simulink model "Final_System_Model_V10"  (R2018a)
settings: Solver=VariableStepAuto  StartTime=0  StopTime=250  FixedStep=0.5  RelTol=1e-3
PreLoadFcn:
  | Ts_Power=1e-6;
  | Ts_Control=100e-6;
undefined symbols (not defined in the file): DiscIntNeverNeededParam, sigbuilder_block
libraries: simulink x24, fl_lib x16, powerlib x15, nesl_utility x8, powerlib_meascontrol x5, re_lib x1
(part 7 of 8)

== system Final_System_Model_V10/Full System/Subsystem1/100KW Fuel Cell Stack_2/Fuel Cell Model/ From Current Density (A//cm^2) To Overvoltages (V)/Activation Overvoltage ==
  note: % Activation Losses
      | b = R .*Tk./(2 .*Alpha .*F);
      | V_act = -b .*log(i./io) % Tafel equation
  Temperature/C1 : Inport
  Current Density (i)(A/cm^2) : Inport  Port=2
  Add : Sum
  Alpha Charge Transfer Coefficient1 : Constant  Value=Alpha_charge_Transfer_Coefficient
  Bus Creator : BusCreator  Inputs=6
  Bus Creator1 : BusCreator  Inputs=3
  Bus Selector : BusSelector  OutputSignals=8:314,Stack Temperature (C),273:15,2,Faraday Constant,Alpha
  Bus Selector1 : BusSelector  OutputSignals=b,Current Density (A/cm^2),i_0
  Constant : Constant  Value=273.15
  Constant1 : Constant  Value=8.314
  Constant2 : Constant  Value=2
  Divide : Product  Inputs=*/
  Farady Constant : Constant  Value=96485
  Gain : Gain  Gain=-1
  Math Function : Math  Operator=log10  SaturateOnIntegerOverflow=on
  Product : Product  Inputs=3
  Product1 : Product
  Product2 : Product
  Reference Exchange Current Density (I_0)1 : Constant  Value=Exchange_Current_Density_i0
  b : Product  Inputs=*/
  Activation Overvoltage1 (V) : Outport
  Exchange Current Density (i_0) : Outport  Port=2
  wires:
  Alpha Charge Transfer Coefficient1/1 -> Bus Creator/2  "Alpha"
  Temperature/C1/1 -> Bus Creator/1
  Current Density (i)(A/cm^2)/1 -> Bus Creator1/2
  Reference Exchange Current Density (I_0)1/1 -> Bus Creator1/3, Exchange Current Density (i_0)/1  "i_0"
  Product2/1 -> Activation Overvoltage1 (V)/1  "Activation Overvoltage"
  Bus Creator/1 -> Bus Selector/1
  Constant/1 -> Bus Creator/3  "273:15"
  Constant1/1 -> Bus Creator/4  "8:314"
  Farady Constant/1 -> Bus Creator/5  "Faraday Constant"
  Constant2/1 -> Bus Creator/6  "2"
  Bus Selector/4 -> Product/1  "<2>"
  Bus Selector/5 -> Product/2  "<Faraday Constant>"
  Bus Selector/6 -> Product/3  "<Alpha>"
  Product/1 -> b/2
  Bus Selector/1 -> Product1/1  "<8:314>"
  Bus Selector/2 -> Add/1  "<Stack Temperature (C)>"
  Bus Selector/3 -> Add/2  "<273:15>"
  Add/1 -> Product1/2  "Temperature/K"
  Product1/1 -> b/1
  b/1 -> Bus Creator1/1  "b"
  Bus Creator1/1 -> Bus Selector1/1
  Bus Selector1/1 -> Gain/1  "<b>"
  Bus Selector1/2 -> Divide/1  "<Current Density (A/cm^2)>"
  Bus Selector1/3 -> Divide/2  "<i_0>"
  Gain/1 -> Product2/1
  Divide/1 -> Math Function/1
  Math Function/1 -> Product2/2

== system Final_System_Model_V10/Full System/Subsystem1/100KW Fuel Cell Stack_2/Fuel Cell Model/ From Current Density (A//cm^2) To Overvoltages (V)/Concentration Overvoltage ==
  note: V_conc = Alpha1 .*(i.^k) .*log(1-(i./il));
      | term=1-(i/i_l)
  Current Density (i)1 : Inport
  Add : Sum  Inputs=+-
  Amplification Constant Alpha2 : Constant  Value=Amplification_Constant_Alpha1
  Bus Creator : BusCreator  Inputs=3
  Bus Creator1 : BusCreator  Inputs=4
  Bus Selector : BusSelector  OutputSignals=1,Current Density (i),Limiting Current Density (i_L)
  Bus Selector1 : BusSelector  OutputSignals=Amplification Constant(Alpha1),Current Density (i),Mass Transport Limit (K),ln term
  Constant : Constant
  Constant1 : Constant  Value=0.01
  Constant2 : Constant  Value=0
  Divide : Product  Inputs=*/
  IF Function : Subsystem
  Limiting Current (i_L)1 : Constant  Value=Limiting_Current_Density_i_l
  Mass Transport Constant (K)1 : Constant  Value=Mass_Transport_Limit_k
  Math Function1 : Math  Operator=pow  SaturateOnIntegerOverflow=on
  Product : Product  Inputs=3
  Saturation Dynamic : simulink/Discontinuities/Saturation Dynamic  OutMin=[]  OutMax=[]  OutDataTypeStr=Inherit: Same as second input  OutDataType=fixdt(1, 16)  OutScaling=2^-10  DoSatur=off
  Subtract : Sum  Inputs=+-
  "Concentration Overvoltage1 (V) " : Outport
  wires:
  Bus Creator/1 -> Bus Selector/1
  Limiting Current (i_L)1/1 -> Subtract/1, Bus Creator/2  "Limiting Current Density (i_L)"
  Saturation Dynamic/1 -> Bus Creator1/1, Bus Creator/1  "Current Density (i)"
  Mass Transport Constant (K)1/1 -> Bus Creator1/2  "Mass Transport Limit (K)"
  Amplification Constant Alpha2/1 -> Bus Creator1/4  "Amplification Constant(Alpha1)"
  Product/1 -> "Concentration Overvoltage1 (V) "/1  "Concentration Overvoltage"
  Constant/1 -> Bus Creator/3  "1"
  Bus Selector/1 -> Add/1  "<1>"
  Bus Selector/2 -> Divide/1  "<Current Density (i)>"
  Bus Selector/3 -> Divide/2  "<Limiting Current Density (i_L)>"
  Divide/1 -> Add/2
  Add/1 -> IF Function/1(In1)
  IF Function/1(Out1) -> Bus Creator1/3  "ln term"
  Bus Creator1/1 -> Bus Selector1/1
  Bus Selector1/1 -> Product/1  "<Amplification Constant(Alpha1)>"
  Bus Selector1/2 -> Math Function1/1  "<Current Density (i)>"
  Bus Selector1/3 -> Math Function1/2  "<Mass Transport Limit (K)>"
  Bus Selector1/4 -> Product/3  "<ln term>"
  Math Function1/1 -> Product/2
  Current Density (i)1/1 -> Saturation Dynamic/2  "Current Density (i)"
  Constant1/1 -> Subtract/2
  Subtract/1 -> Saturation Dynamic/1
  Constant2/1 -> Saturation Dynamic/3

== system Final_System_Model_V10/Full System/Subsystem1/100KW Fuel Cell Stack_2/Fuel Cell Model/ From Current Density (A//cm^2) To Overvoltages (V)/Ohmic Overvoltage ==
  Current Density (i ) : Inport
  Constant : Constant  Value=-1
  Internal Resistance (r) : Constant  Value=Internal_Resistance_r
  V_Resistive1 : Product  Inputs=3
  V_Resistive : Outport
  wires:
  Constant/1 -> V_Resistive1/3
  Internal Resistance (r)/1 -> V_Resistive1/2
  Current Density (i )/1 -> V_Resistive1/1
  V_Resistive1/1 -> V_Resistive/1  "Ohmic Overvoltage (V)"

== system Final_System_Model_V10/Full System/Subsystem1/100KW Fuel Cell Stack_2/Fuel Cell Model/Air Flow Rate To Current (A)/From Stack Current (A) To Oxygen Mass Flow Rate(kg//s) ==
  Current (A) : Inport
  Number Of Cells : Inport  Port=2
  Divide : Product  Inputs=*/
  F : Constant  Value=96487
  Oxygen Molar Mass (Kg/mol) : Constant  Value=32e-3
  Product : Product
  Product1 : Product
  Product2 : Product
  c : Constant  Value=4
  Oxygen Flow Rate (kg/s) : Outport
  wires:
  F/1 -> Product1/1
  Current (A)/1 -> Product/1
  Product/1 -> Divide/1
  Oxygen Molar Mass (Kg/mol)/1 -> Product2/2
  c/1 -> Product1/2
  Divide/1 -> Product2/1
  Product1/1 -> Divide/2
  Product2/1 -> Oxygen Flow Rate (kg/s)/1
  Number Of Cells/1 -> Product/2

== system Final_System_Model_V10/Full System/Subsystem1/100KW Fuel Cell Stack_2/Fuel Cell Model/From Mass Flow Rates (kg//s) To Current Density (A//cm^2)/From Current (A) To Current Density (A//cm^2) ==
  note: i=I/A
      | where i=Current Density (A/cm^2)
      | I= Current (A)
      | A=Cell Area (cm^2)
  Nominal Current (A) : Inport
  Cell Area (cm^2) : Inport  Port=2
  Divide : Product  Inputs=*/
  Current Density (A/cm^2) : Outport
  wires:
  Nominal Current (A)/1 -> Divide/1
  Cell Area (cm^2)/1 -> Divide/2
  Divide/1 -> Current Density (A/cm^2)/1

== system Final_System_Model_V10/Full System/Subsystem1/100KW Fuel Cell Stack_2/Fuel Cell Model/From Mass Flow Rates (kg//s) To Current Density (A//cm^2)/Fuel Mass Flow Rate (kg//s) To Current (A) ==
  note: This block calculates the output Current (A) from the Hydrogen Mass Flow Rate (kg/s)
      | I=Hydrogen Mass Flow Rate (kg/s)*2*F/(M_H2*n)
      | where: I=Current (A)
      | F=Faraday Constant=96487 C/mol
      | M_H2=hydrogen molar mass=2.016*10^-3 kg/mol
      | n=Number of Cells
  Hydrogen Flow Rate (kg/s) : Inport
  Number Of Cells : Inport  Port=2
  Constant1 : Constant  Value=2
  Divide : Product  Inputs=*/
  F : Constant  Value=96487
  Hydrogen Molar Mass : Constant  Value=2.016e-3
  Product : Product
  Product1 : Product
  Product2 : Product
  Current (A) : Outport
  wires:
  F/1 -> Product1/2
  Constant1/1 -> Product1/1
  Product1/1 -> Product/2
  Product/1 -> Divide/1
  Hydrogen Molar Mass/1 -> Product2/1
  Number Of Cells/1 -> Product2/2
  Product2/1 -> Divide/2
  Divide/1 -> Current (A)/1
  Hydrogen Flow Rate (kg/s)/1 -> Product/1

== system Final_System_Model_V10/Full System/Subsystem1/100KW Fuel Cell Stack_2/Fuel Cell Model/From Pressures (atm) To Nernest Voltage (V)/From Absolute Pressure (atm) To Partial Pressures (atm) ==
  Current Density (i ) : Inport
  Hydrogen Pressure (P_H2) : Inport  Port=2
  Air Pressure (P_air) : Inport  Port=3
  Temperature/C : Inport  Port=4
  Bus Creator : BusCreator  Inputs=5
  Bus Selector : BusSelector  OutputSignals=Air Pressure (atm),Stack Temperature (C),Current Density (A/cm^2),Water Pressure(atm)
  Bus Selector1 : BusSelector  OutputSignals=Stack Temperature (C)
  Bus Selector2 : BusSelector  OutputSignals=Hydrogen Pressure (atm),Stack Temperature (C),Current Density (A/cm^2),Water Pressure(atm)
  Hydrogen Partial Pressure Output : Subsystem
  Oxygen Partial Pressure Output : Subsystem
  Water Pressure output : Subsystem
  Hydrogen Partial Pressure (pp_H2) : Outport
  Oxygen Partial Pressure pp_O2 : Outport  Port=2
  Water Pressure : Outport  Port=3
  wires:
  Water Pressure output/1(Water Pressure) -> Water Pressure/1, Bus Creator/3
  Air Pressure (P_air)/1 -> Bus Creator/1
  Oxygen Partial Pressure Output/1(Oxygen Partial Pressure pp_O2) -> Oxygen Partial Pressure pp_O2/1
  Hydrogen Partial Pressure Output/1(Hydrogen Partial Pressure (pp_H2)) -> Hydrogen Partial Pressure (pp_H2)/1
  Current Density (i )/1 -> Bus Creator/2  "Current Density (A/cm^2)"
  Temperature/C/1 -> Bus Creator/4
  Hydrogen Pressure (P_H2)/1 -> Bus Creator/5
  Bus Creator/1 -> Bus Selector2/1, Bus Selector/1, Bus Selector1/1
  Bus Selector/1 -> Oxygen Partial Pressure Output/1(Air Pressure (P_air))  "<Air Pressure (atm)>"
  Bus Selector/2 -> Oxygen Partial Pressure Output/2(Temperature/C)  "<Stack Temperature (C)>"
  Bus Selector/3 -> Oxygen Partial Pressure Output/3(Current Density/i)  "<Current Density (A/cm^2)>"
  Bus Selector/4 -> Oxygen Partial Pressure Output/4(Water Pressure)  "<Water Pressure(atm)>"
  Bus Selector1/1 -> Water Pressure output/1(Temperature/C)  "<Stack Temperature (C)>"
  Bus Selector2/1 -> Hydrogen Partial Pressure Output/1(Hydrogen Pressure (P_H2))  "<Hydrogen Pressure (atm)>"
  Bus Selector2/2 -> Hydrogen Partial Pressure Output/2(Temperature/C)  "<Stack Temperature (C)>"
  Bus Selector2/3 -> Hydrogen Partial Pressure Output/3(Current Density (i ))  "<Current Density (A/cm^2)>"
  Bus Selector2/4 -> Hydrogen Partial Pressure Output/4(Water Pressure)  "<Water Pressure(atm)>"

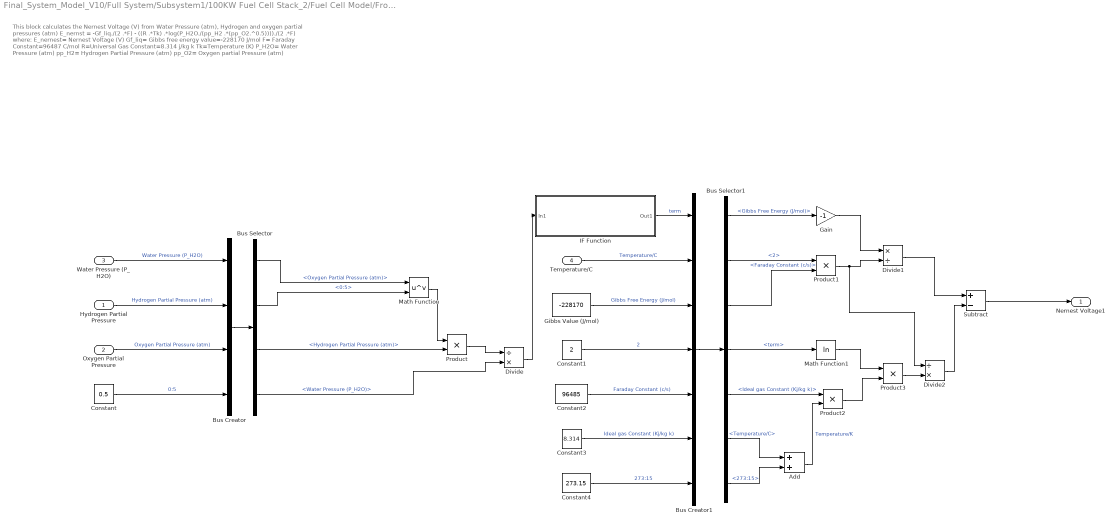
== system Final_System_Model_V10/Full System/Subsystem1/100KW Fuel Cell Stack_2/Fuel Cell Model/From Pressures (atm) To Nernest Voltage (V)/From Partial Pressures (atm) To Nernest Voltage (V) ==
  note: This block calculates the Nernest Voltage (V) from Water Pressure (atm), Hydrogen and oxygen partial pressures (atm)
      | E_nernst = -Gf_liq./(2 .*F) - ((R .*Tk) .*log(P_H2O./(pp_H2 .*(pp_O2.^0.5))))./(2 .*F)
      | where: E_nernest= Nernest Voltage (V)
      | Gf_liq= Gibbs free energy value=-228170 J/mol
      | F= Faraday Constant=96487 C/mol
      | R=Universal Gas Constant=8.314 j/kg k
      | Tk=Temperature (K)
      | P_H2O= Water Pressure (atm)
      | pp_H2= Hydrogen Partial Pressure (atm)
      | pp_O2= Oxygen partial Pressure (atm)
  Hydrogen Partial Pressure : Inport
  Oxygen Partial Pressure : Inport  Port=2
  Water Pressure (P_H2O) : Inport  Port=3
  Temperature/C : Inport  Port=4
  Add : Sum
  Bus Creator : BusCreator  Inputs=4
  Bus Creator1 : BusCreator  Inputs=7
  Bus Selector : BusSelector  OutputSignals=Oxygen Partial Pressure (atm),0:5,Hydrogen Partial Pressure (atm),Water Pressure (P_H2O)
  Bus Selector1 : BusSelector  OutputSignals=Gibbs Free Energy (J/mol),2,Faraday Constant (c/s),term,Ideal gas Constant (Kj/kg k),Temperature/C,273:15
  Constant : Constant  Value=0.5
  Constant1 : Constant  Value=2
  Constant2 : Constant  Value=96485
  Constant3 : Constant  Value=8.314
  Constant4 : Constant  Value=273.15
  Divide : Product  Inputs=/*
  Divide1 : Product  Inputs=*/
  Divide2 : Product  Inputs=/*
  Gain : Gain  Gain=-1
  Gibbs Value (J/mol) : Constant  Value=-228170
  IF Function : Subsystem
  Math Function : Math  Operator=pow  SaturateOnIntegerOverflow=on
  Math Function1 : Math  Operator=log  SaturateOnIntegerOverflow=on
  Product{,1..3} (4 alike) : Product
  Subtract : Sum  Inputs=+-
  Nernest Voltage1 : Outport
  wires:
  Gibbs Value (J/mol)/1 -> Bus Creator1/3  "Gibbs Free Energy (J/mol)"
  Oxygen Partial Pressure/1 -> Bus Creator/3  "Oxygen Partial Pressure (atm)"
  Water Pressure (P_H2O)/1 -> Bus Creator/1  "Water Pressure (P_H2O)"
  Hydrogen Partial Pressure/1 -> Bus Creator/2  "Hydrogen Partial Pressure (atm)"
  Temperature/C/1 -> Bus Creator1/2  "Temperature/C"
  Bus Creator/1 -> Bus Selector/1
  Bus Selector/2 -> Math Function/2  "<0:5>"
  Constant/1 -> Bus Creator/4  "0:5"
  Bus Selector/1 -> Math Function/1  "<Oxygen Partial Pressure (atm)>"
  Bus Selector/3 -> Product/2  "<Hydrogen Partial Pressure (atm)>"
  Math Function/1 -> Product/1
  Bus Selector/4 -> Divide/2  "<Water Pressure (P_H2O)>"
  Product/1 -> Divide/1
  Divide/1 -> IF Function/1(In1)
  IF Function/1(Out1) -> Bus Creator1/1  "term"
  Bus Creator1/1 -> Bus Selector1/1
  Constant1/1 -> Bus Creator1/4  "2"
  Constant2/1 -> Bus Creator1/5  "Faraday Constant (c/s)"
  Bus Selector1/1 -> Gain/1  "<Gibbs Free Energy (J/mol)>"
  Gain/1 -> Divide1/1
  Bus Selector1/2 -> Product1/1  "<2>"
  Bus Selector1/3 -> Product1/2  "<Faraday Constant (c/s)>"
  Product1/1 -> Divide2/1, Divide1/2
  Divide1/1 -> Subtract/1
  Bus Selector1/4 -> Math Function1/1  "<term>"
  Math Function1/1 -> Product3/1
  Constant3/1 -> Bus Creator1/6  "Ideal gas Constant (Kj/kg k)"
  Constant4/1 -> Bus Creator1/7  "273:15"
  Bus Selector1/5 -> Product2/1  "<Ideal gas Constant (Kj/kg k)>"
  Bus Selector1/6 -> Add/1  "<Temperature/C>"
  Bus Selector1/7 -> Add/2  "<273:15>"
  Add/1 -> Product2/2  "Temperature/K"
  Product2/1 -> Product3/2
  Product3/1 -> Divide2/2
  Divide2/1 -> Subtract/2
  Subtract/1 -> Nernest Voltage1/1

== system Final_System_Model_V10/Full System/Subsystem1/80KW Fuel Cell Stack_1/Fuel Cell Model/ From Current Density (A//cm^2) To Overvoltages (V)/Activation Overvoltage ==
  note: % Activation Losses
      | b = R .*Tk./(2 .*Alpha .*F);
      | V_act = -b .*log(i./io) % Tafel equation
  Temperature/C1 : Inport
  Current Density (i)(A/cm^2) : Inport  Port=2
  Add : Sum
  Alpha Charge Transfer Coefficient1 : Constant  Value=Alpha_charge_Transfer_Coefficient
  Bus Creator : BusCreator  Inputs=6
  Bus Creator1 : BusCreator  Inputs=3
  Bus Selector : BusSelector  OutputSignals=8:314,Stack Temperature (C),273:15,2,Faraday Constant,Alpha
  Bus Selector1 : BusSelector  OutputSignals=b,Current Density (A/cm^2),i_0
  Constant : Constant  Value=273.15
  Constant1 : Constant  Value=8.314
  Constant2 : Constant  Value=2
  Divide : Product  Inputs=*/
  Farady Constant : Constant  Value=96485
  Gain : Gain  Gain=-1
  Math Function : Math  Operator=log10  SaturateOnIntegerOverflow=on
  Product : Product  Inputs=3
  Product1 : Product
  Product2 : Product
  Reference Exchange Current Density (I_0)1 : Constant  Value=Exchange_Current_Density_i0
  b : Product  Inputs=*/
  Activation Overvoltage1 (V) : Outport
  Exchange Current Density (i_0) : Outport  Port=2
  wires:
  Math Function/1 -> Product2/2
  Divide/1 -> Math Function/1
  Gain/1 -> Product2/1
  Bus Selector1/3 -> Divide/2  "<i_0>"
  Bus Selector1/2 -> Divide/1  "<Current Density (A/cm^2)>"
  Bus Selector1/1 -> Gain/1  "<b>"
  Bus Creator1/1 -> Bus Selector1/1
  b/1 -> Bus Creator1/1  "b"
  Product1/1 -> b/1
  Add/1 -> Product1/2  "Temperature/K"
  Bus Selector/3 -> Add/2  "<273:15>"
  Bus Selector/2 -> Add/1  "<Stack Temperature (C)>"
  Bus Selector/1 -> Product1/1  "<8:314>"
  Product/1 -> b/2
  Bus Selector/6 -> Product/3  "<Alpha>"
  Bus Selector/5 -> Product/2  "<Faraday Constant>"
  Bus Selector/4 -> Product/1  "<2>"
  Constant2/1 -> Bus Creator/6  "2"
  Farady Constant/1 -> Bus Creator/5  "Faraday Constant"
  Constant1/1 -> Bus Creator/4  "8:314"
  Constant/1 -> Bus Creator/3  "273:15"
  Bus Creator/1 -> Bus Selector/1
  Product2/1 -> Activation Overvoltage1 (V)/1  "Activation Overvoltage"
  Reference Exchange Current Density (I_0)1/1 -> Exchange Current Density (i_0)/1, Bus Creator1/3  "i_0"
  Current Density (i)(A/cm^2)/1 -> Bus Creator1/2
  Temperature/C1/1 -> Bus Creator/1
  Alpha Charge Transfer Coefficient1/1 -> Bus Creator/2  "Alpha"

== system Final_System_Model_V10/Full System/Subsystem1/80KW Fuel Cell Stack_1/Fuel Cell Model/ From Current Density (A//cm^2) To Overvoltages (V)/Concentration Overvoltage ==
  note: V_conc = Alpha1 .*(i.^k) .*log(1-(i./il));
      | term=1-(i/i_l)
  Current Density (i)1 : Inport
  Add : Sum  Inputs=+-
  Amplification Constant Alpha2 : Constant  Value=Amplification_Constant_Alpha1
  Bus Creator : BusCreator  Inputs=3
  Bus Creator1 : BusCreator  Inputs=4
  Bus Selector : BusSelector  OutputSignals=1,Current Density (i),Limiting Current Density (i_L)
  Bus Selector1 : BusSelector  OutputSignals=Amplification Constant(Alpha1),Current Density (i),Mass Transport Limit (K),ln term
  Constant : Constant
  Constant1 : Constant  Value=0.01
  Constant2 : Constant  Value=0
  Divide : Product  Inputs=*/
  IF Function : Subsystem
  Limiting Current (i_L)1 : Constant  Value=Limiting_Current_Density_i_l
  Mass Transport Constant (K)1 : Constant  Value=Mass_Transport_Limit_k
  Math Function1 : Math  Operator=pow  SaturateOnIntegerOverflow=on
  Product : Product  Inputs=3
  Saturation Dynamic : simulink/Discontinuities/Saturation Dynamic  OutMin=[]  OutMax=[]  OutDataTypeStr=Inherit: Same as second input  OutDataType=fixdt(1, 16)  OutScaling=2^-10  DoSatur=off
  Subtract : Sum  Inputs=+-
  "Concentration Overvoltage1 (V) " : Outport
  wires:
  Constant2/1 -> Saturation Dynamic/3
  Subtract/1 -> Saturation Dynamic/1
  Constant1/1 -> Subtract/2
  Current Density (i)1/1 -> Saturation Dynamic/2  "Current Density (i)"
  Math Function1/1 -> Product/2
  Bus Selector1/4 -> Product/3  "<ln term>"
  Bus Selector1/3 -> Math Function1/2  "<Mass Transport Limit (K)>"
  Bus Selector1/2 -> Math Function1/1  "<Current Density (i)>"
  Bus Selector1/1 -> Product/1  "<Amplification Constant(Alpha1)>"
  Bus Creator1/1 -> Bus Selector1/1
  IF Function/1(Out1) -> Bus Creator1/3  "ln term"
  Add/1 -> IF Function/1(In1)
  Divide/1 -> Add/2
  Bus Selector/3 -> Divide/2  "<Limiting Current Density (i_L)>"
  Bus Selector/2 -> Divide/1  "<Current Density (i)>"
  Bus Selector/1 -> Add/1  "<1>"
  Constant/1 -> Bus Creator/3  "1"
  Product/1 -> "Concentration Overvoltage1 (V) "/1  "Concentration Overvoltage"
  Amplification Constant Alpha2/1 -> Bus Creator1/4  "Amplification Constant(Alpha1)"
  Mass Transport Constant (K)1/1 -> Bus Creator1/2  "Mass Transport Limit (K)"
  Saturation Dynamic/1 -> Bus Creator/1, Bus Creator1/1  "Current Density (i)"
  Limiting Current (i_L)1/1 -> Bus Creator/2, Subtract/1  "Limiting Current Density (i_L)"
  Bus Creator/1 -> Bus Selector/1

== system Final_System_Model_V10/Full System/Subsystem1/80KW Fuel Cell Stack_1/Fuel Cell Model/ From Current Density (A//cm^2) To Overvoltages (V)/Ohmic Overvoltage ==
  Current Density (i ) : Inport
  Constant : Constant  Value=-1
  Internal Resistance (r) : Constant  Value=Internal_Resistance_r
  V_Resistive1 : Product  Inputs=3
  V_Resistive : Outport
  wires:
  V_Resistive1/1 -> V_Resistive/1  "Ohmic Overvoltage (V)"
  Current Density (i )/1 -> V_Resistive1/1
  Internal Resistance (r)/1 -> V_Resistive1/2
  Constant/1 -> V_Resistive1/3

== system Final_System_Model_V10/Full System/Subsystem1/80KW Fuel Cell Stack_1/Fuel Cell Model/Air Flow Rate To Current (A)/From Stack Current (A) To Oxygen Mass Flow Rate(kg//s) ==
  Current (A) : Inport
  Number Of Cells : Inport  Port=2
  Divide : Product  Inputs=*/
  F : Constant  Value=96487
  Oxygen Molar Mass (Kg/mol) : Constant  Value=32e-3
  Product : Product
  Product1 : Product
  Product2 : Product
  c : Constant  Value=4
  Oxygen Flow Rate (kg/s) : Outport
  wires:
  Number Of Cells/1 -> Product/2
  Product2/1 -> Oxygen Flow Rate (kg/s)/1
  Product1/1 -> Divide/2
  Divide/1 -> Product2/1
  c/1 -> Product1/2
  Oxygen Molar Mass (Kg/mol)/1 -> Product2/2
  Product/1 -> Divide/1
  Current (A)/1 -> Product/1
  F/1 -> Product1/1

== system Final_System_Model_V10/Full System/Subsystem1/80KW Fuel Cell Stack_1/Fuel Cell Model/From Mass Flow Rates (kg//s) To Current Density (A//cm^2)/From Current (A) To Current Density (A//cm^2) ==
  note: i=I/A
      | where i=Current Density (A/cm^2)
      | I= Current (A)
      | A=Cell Area (cm^2)
  Nominal Current (A) : Inport
  Cell Area (cm^2) : Inport  Port=2
  Divide : Product  Inputs=*/
  Current Density (A/cm^2) : Outport
  wires:
  Divide/1 -> Current Density (A/cm^2)/1
  Cell Area (cm^2)/1 -> Divide/2
  Nominal Current (A)/1 -> Divide/1

== system Final_System_Model_V10/Full System/Subsystem1/80KW Fuel Cell Stack_1/Fuel Cell Model/From Mass Flow Rates (kg//s) To Current Density (A//cm^2)/Fuel Mass Flow Rate (kg//s) To Current (A) ==
  note: This block calculates the output Current (A) from the Hydrogen Mass Flow Rate (kg/s)
      | I=Hydrogen Mass Flow Rate (kg/s)*2*F/(M_H2*n)
      | where: I=Current (A)
      | F=Faraday Constant=96487 C/mol
      | M_H2=hydrogen molar mass=2.016*10^-3 kg/mol
      | n=Number of Cells
  Hydrogen Flow Rate (kg/s) : Inport
  Number Of Cells : Inport  Port=2
  Constant1 : Constant  Value=2
  Divide : Product  Inputs=*/
  F : Constant  Value=96487
  Hydrogen Molar Mass : Constant  Value=2.016e-3
  Product : Product
  Product1 : Product
  Product2 : Product
  Current (A) : Outport
  wires:
  Hydrogen Flow Rate (kg/s)/1 -> Product/1
  Divide/1 -> Current (A)/1
  Product2/1 -> Divide/2
  Number Of Cells/1 -> Product2/2
  Hydrogen Molar Mass/1 -> Product2/1
  Product/1 -> Divide/1
  Product1/1 -> Product/2
  Constant1/1 -> Product1/1
  F/1 -> Product1/2

== system Final_System_Model_V10/Full System/Subsystem1/80KW Fuel Cell Stack_1/Fuel Cell Model/From Pressures (atm) To Nernest Voltage (V)/From Absolute Pressure (atm) To Partial Pressures (atm) ==
  Current Density (i ) : Inport
  Hydrogen Pressure (P_H2) : Inport  Port=2
  Air Pressure (P_air) : Inport  Port=3
  Temperature/C : Inport  Port=4
  Bus Creator : BusCreator  Inputs=5
  Bus Selector : BusSelector  OutputSignals=Air Pressure (atm),Stack Temperature (C),Current Density (A/cm^2),Water Pressure(atm)
  Bus Selector1 : BusSelector  OutputSignals=Stack Temperature (C)
  Bus Selector2 : BusSelector  OutputSignals=Hydrogen Pressure (atm),Stack Temperature (C),Current Density (A/cm^2),Water Pressure(atm)
  Hydrogen Partial Pressure Output : Subsystem
  Oxygen Partial Pressure Output : Subsystem
  Water Pressure output : Subsystem
  Hydrogen Partial Pressure (pp_H2) : Outport
  Oxygen Partial Pressure pp_O2 : Outport  Port=2
  Water Pressure : Outport  Port=3
  wires:
  Bus Selector2/4 -> Hydrogen Partial Pressure Output/4(Water Pressure)  "<Water Pressure(atm)>"
  Bus Selector2/3 -> Hydrogen Partial Pressure Output/3(Current Density (i ))  "<Current Density (A/cm^2)>"
  Bus Selector2/2 -> Hydrogen Partial Pressure Output/2(Temperature/C)  "<Stack Temperature (C)>"
  Bus Selector2/1 -> Hydrogen Partial Pressure Output/1(Hydrogen Pressure (P_H2))  "<Hydrogen Pressure (atm)>"
  Bus Selector1/1 -> Water Pressure output/1(Temperature/C)  "<Stack Temperature (C)>"
  Bus Selector/4 -> Oxygen Partial Pressure Output/4(Water Pressure)  "<Water Pressure(atm)>"
  Bus Selector/3 -> Oxygen Partial Pressure Output/3(Current Density/i)  "<Current Density (A/cm^2)>"
  Bus Selector/2 -> Oxygen Partial Pressure Output/2(Temperature/C)  "<Stack Temperature (C)>"
  Bus Selector/1 -> Oxygen Partial Pressure Output/1(Air Pressure (P_air))  "<Air Pressure (atm)>"
  Bus Creator/1 -> Bus Selector1/1, Bus Selector/1, Bus Selector2/1
  Hydrogen Pressure (P_H2)/1 -> Bus Creator/5
  Temperature/C/1 -> Bus Creator/4
  Current Density (i )/1 -> Bus Creator/2  "Current Density (A/cm^2)"
  Hydrogen Partial Pressure Output/1(Hydrogen Partial Pressure (pp_H2)) -> Hydrogen Partial Pressure (pp_H2)/1
  Oxygen Partial Pressure Output/1(Oxygen Partial Pressure pp_O2) -> Oxygen Partial Pressure pp_O2/1
  Air Pressure (P_air)/1 -> Bus Creator/1
  Water Pressure output/1(Water Pressure) -> Bus Creator/3, Water Pressure/1

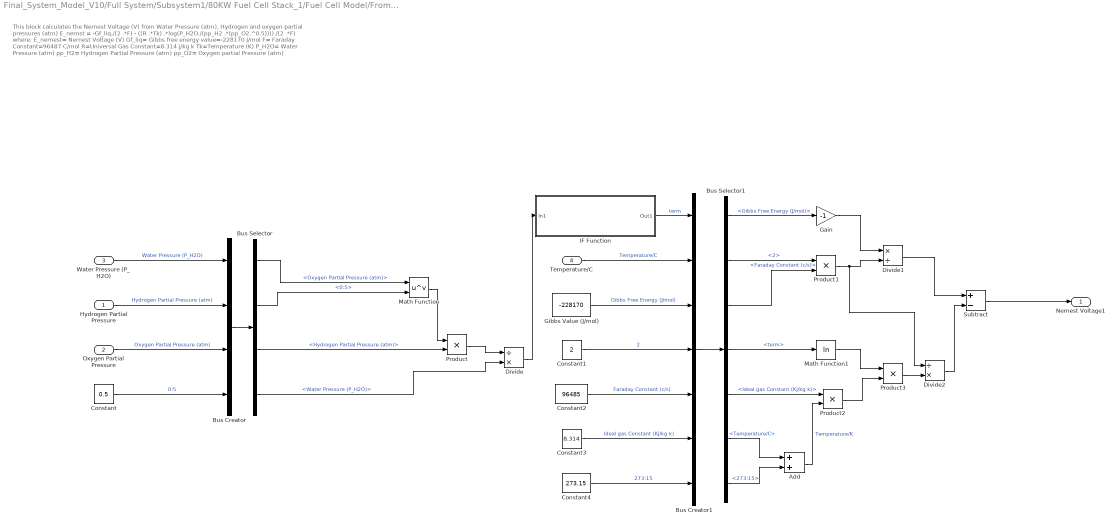
== system Final_System_Model_V10/Full System/Subsystem1/80KW Fuel Cell Stack_1/Fuel Cell Model/From Pressures (atm) To Nernest Voltage (V)/From Partial Pressures (atm) To Nernest Voltage (V) ==
  note: This block calculates the Nernest Voltage (V) from Water Pressure (atm), Hydrogen and oxygen partial pressures (atm)
      | E_nernst = -Gf_liq./(2 .*F) - ((R .*Tk) .*log(P_H2O./(pp_H2 .*(pp_O2.^0.5))))./(2 .*F)
      | where: E_nernest= Nernest Voltage (V)
      | Gf_liq= Gibbs free energy value=-228170 J/mol
      | F= Faraday Constant=96487 C/mol
      | R=Universal Gas Constant=8.314 j/kg k
      | Tk=Temperature (K)
      | P_H2O= Water Pressure (atm)
      | pp_H2= Hydrogen Partial Pressure (atm)
      | pp_O2= Oxygen partial Pressure (atm)
  Hydrogen Partial Pressure : Inport
  Oxygen Partial Pressure : Inport  Port=2
  Water Pressure (P_H2O) : Inport  Port=3
  Temperature/C : Inport  Port=4
  Add : Sum
  Bus Creator : BusCreator  Inputs=4
  Bus Creator1 : BusCreator  Inputs=7
  Bus Selector : BusSelector  OutputSignals=Oxygen Partial Pressure (atm),0:5,Hydrogen Partial Pressure (atm),Water Pressure (P_H2O)
  Bus Selector1 : BusSelector  OutputSignals=Gibbs Free Energy (J/mol),2,Faraday Constant (c/s),term,Ideal gas Constant (Kj/kg k),Temperature/C,273:15
  Constant : Constant  Value=0.5
  Constant1 : Constant  Value=2
  Constant2 : Constant  Value=96485
  Constant3 : Constant  Value=8.314
  Constant4 : Constant  Value=273.15
  Divide : Product  Inputs=/*
  Divide1 : Product  Inputs=*/
  Divide2 : Product  Inputs=/*
  Gain : Gain  Gain=-1
  Gibbs Value (J/mol) : Constant  Value=-228170
  IF Function : Subsystem
  Math Function : Math  Operator=pow  SaturateOnIntegerOverflow=on
  Math Function1 : Math  Operator=log  SaturateOnIntegerOverflow=on
  Product{,1..3} (4 alike) : Product
  Subtract : Sum  Inputs=+-
  Nernest Voltage1 : Outport
  wires:
  Subtract/1 -> Nernest Voltage1/1
  Divide2/1 -> Subtract/2
  Product3/1 -> Divide2/2
  Product2/1 -> Product3/2
  Add/1 -> Product2/2  "Temperature/K"
  Bus Selector1/7 -> Add/2  "<273:15>"
  Bus Selector1/6 -> Add/1  "<Temperature/C>"
  Bus Selector1/5 -> Product2/1  "<Ideal gas Constant (Kj/kg k)>"
  Constant4/1 -> Bus Creator1/7  "273:15"
  Constant3/1 -> Bus Creator1/6  "Ideal gas Constant (Kj/kg k)"
  Math Function1/1 -> Product3/1
  Bus Selector1/4 -> Math Function1/1  "<term>"
  Divide1/1 -> Subtract/1
  Product1/1 -> Divide1/2, Divide2/1
  Bus Selector1/3 -> Product1/2  "<Faraday Constant (c/s)>"
  Bus Selector1/2 -> Product1/1  "<2>"
  Gain/1 -> Divide1/1
  Bus Selector1/1 -> Gain/1  "<Gibbs Free Energy (J/mol)>"
  Constant2/1 -> Bus Creator1/5  "Faraday Constant (c/s)"
  Constant1/1 -> Bus Creator1/4  "2"
  Bus Creator1/1 -> Bus Selector1/1
  IF Function/1(Out1) -> Bus Creator1/1  "term"
  Divide/1 -> IF Function/1(In1)
  Product/1 -> Divide/1
  Bus Selector/4 -> Divide/2  "<Water Pressure (P_H2O)>"
  Math Function/1 -> Product/1
  Bus Selector/3 -> Product/2  "<Hydrogen Partial Pressure (atm)>"
  Bus Selector/1 -> Math Function/1  "<Oxygen Partial Pressure (atm)>"
  Constant/1 -> Bus Creator/4  "0:5"
  Bus Selector/2 -> Math Function/2  "<0:5>"
  Bus Creator/1 -> Bus Selector/1
  Temperature/C/1 -> Bus Creator1/2  "Temperature/C"
  Hydrogen Partial Pressure/1 -> Bus Creator/2  "Hydrogen Partial Pressure (atm)"
  Water Pressure (P_H2O)/1 -> Bus Creator/1  "Water Pressure (P_H2O)"
  Oxygen Partial Pressure/1 -> Bus Creator/3  "Oxygen Partial Pressure (atm)"
  Gibbs Value (J/mol)/1 -> Bus Creator1/3  "Gibbs Free Energy (J/mol)"

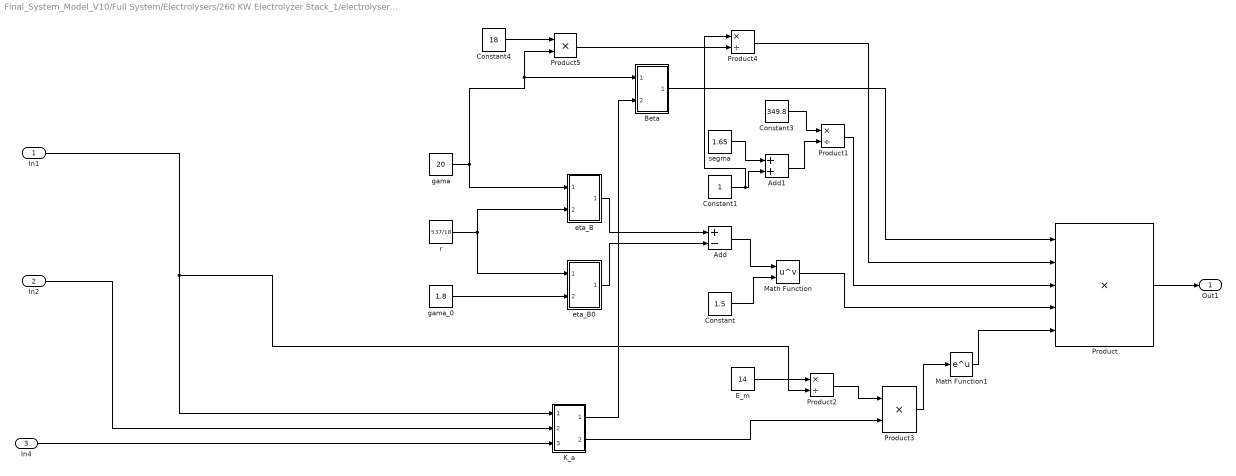
== system Final_System_Model_V10/Full System/Electrolysers/260 KW Electrolyzer Stack_1/electrolyser stack/electrolyser cell/Eta_B/segma_B ==
  In1 : Inport
  In2 : Inport  Port=2
  In4 : Inport  Port=3
  Add : Sum  Inputs=+-
  Add1 : Sum
  Beta : Subsystem
  Constant : Constant  Value=1.5
  Constant1 : Constant
  Constant3 : Constant  Value=349.8
  Constant4 : Constant  Value=18
  E_m : Constant  Value=14
  K_a : Subsystem
  Math Function : Math  Operator=pow  SaturateOnIntegerOverflow=on
  Math Function1 : Math  SaturateOnIntegerOverflow=on
  Product : Product  Inputs=5
  Product1 : Product  Inputs=*/
  Product2 : Product  Inputs=*/
  Product3 : Product
  Product4 : Product  Inputs=*/
  Product5 : Product  Inputs=**
  eta_B : Subsystem
  eta_B0 : Subsystem
  gama : Constant  Value=20
  gama_0 : Constant  Value=1.8
  r : Constant  Value=537/18
  segma : Constant  Value=1.65
  Out1 : Outport
  wires:
  Constant1/1 -> Product4/1, Add1/2
  Math Function1/1 -> Product/5
  eta_B0/1(Out1) -> Add/2
  In4/1 -> K_a/3(In3)
  In1/1 -> Product2/2, K_a/1(In1)
  In2/1 -> K_a/2(In2)
  Product5/1 -> Product4/2
  K_a/1(Out1) -> Beta/2(In2)
  Constant3/1 -> Product1/1
  Math Function/1 -> Product/4
  E_m/1 -> Product2/1
  Constant/1 -> Math Function/2
  Add1/1 -> Product1/2
  segma/1 -> Add1/1
  Product1/1 -> Product/3
  gama_0/1 -> eta_B0/2(In2)
  Product3/1 -> Math Function1/1
  Add/1 -> Math Function/1
  Beta/1(Out1) -> Product/1
  Constant4/1 -> Product5/1
  Product4/1 -> Product/2
  gama/1 -> Product5/2, Beta/1(In1), eta_B/1(In1)
  r/1 -> eta_B0/1(In1), eta_B/2(In2)
  Product/1 -> Out1/1
  eta_B/1(Out1) -> Add/1
  K_a/2(Out2) -> Product3/2
  Product2/1 -> Product3/1

== system Final_System_Model_V10/Full System/Electrolysers/260 KW Electrolyzer Stack_1/electrolyser stack/electrolyser cell/eta_a/m_a ==
  In1 : Inport
  Constant : Constant
  Divide : Product  Inputs=*/
  Subtract : Sum  Inputs=+-
  limiting current : Constant  Value=2
  Out1 : Outport
  wires:
  In1/1 -> Divide/1
  limiting current/1 -> Divide/2
  Constant/1 -> Subtract/1
  Subtract/1 -> Out1/1
  Divide/1 -> Subtract/2

== system Final_System_Model_V10/Full System/Electrolysers/260 KW Electrolyzer Stack_1/electrolyser stack/electrolyser cell/eta_a/n_a ==
  In1 : Inport
  In2 : Inport  Port=2
  In3 : Inport  Port=3
  Divide : Product  Inputs=*/
  i_a0 : Subsystem
  Out1 : Outport
  wires:
  In2/1 -> i_a0/1(In1)
  i_a0/1(Out1) -> Divide/2
  Divide/1 -> Out1/1
  In1/1 -> i_a0/2(In2)
  In3/1 -> Divide/1

== system Final_System_Model_V10/Full System/Electrolysers/260 KW Electrolyzer Stack_1/electrolyser stack/electrolyser cell/eta_c/m_c ==
  In1 : Inport
  Constant : Constant
  Divide : Product  Inputs=*/
  Subtract : Sum  Inputs=+-
  limiting current : Constant  Value=0.00023
  Out1 : Outport
  wires:
  Constant/1 -> Subtract/1
  Subtract/1 -> Out1/1
  limiting current/1 -> Divide/2
  Divide/1 -> Subtract/2
  In1/1 -> Divide/1

== system Final_System_Model_V10/Full System/Electrolysers/260 KW Electrolyzer Stack_1/electrolyser stack/electrolyser cell/eta_c/n_c ==
  In1 : Inport
  In2 : Inport  Port=2
  In3 : Inport  Port=3
  Divide : Product  Inputs=*/
  i_c0 : Subsystem
  Out1 : Outport
  wires:
  In2/1 -> i_c0/1(In1)
  i_c0/1(Out1) -> Divide/2
  In1/1 -> i_c0/2(In2)
  Divide/1 -> Out1/1
  In3/1 -> Divide/1

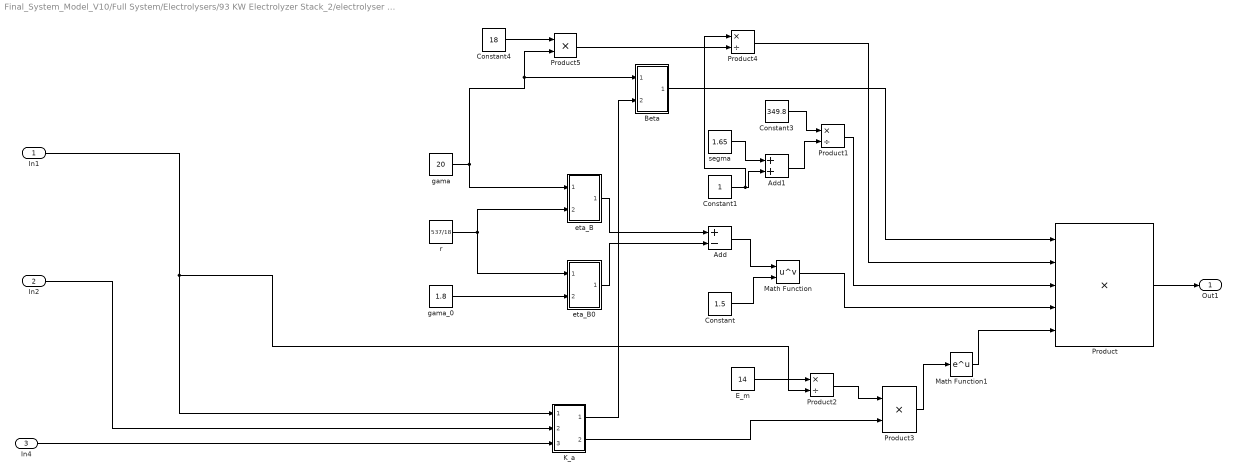
== system Final_System_Model_V10/Full System/Electrolysers/93 KW Electrolyzer Stack_2/electrolyser stack/electrolyser cell/Eta_B/segma_B ==
  In1 : Inport
  In2 : Inport  Port=2
  In4 : Inport  Port=3
  Add : Sum  Inputs=+-
  Add1 : Sum
  Beta : Subsystem
  Constant : Constant  Value=1.5
  Constant1 : Constant
  Constant3 : Constant  Value=349.8
  Constant4 : Constant  Value=18
  E_m : Constant  Value=14
  K_a : Subsystem
  Math Function : Math  Operator=pow  SaturateOnIntegerOverflow=on
  Math Function1 : Math  SaturateOnIntegerOverflow=on
  Product : Product  Inputs=5
  Product1 : Product  Inputs=*/
  Product2 : Product  Inputs=*/
  Product3 : Product
  Product4 : Product  Inputs=*/
  Product5 : Product  Inputs=**
  eta_B : Subsystem
  eta_B0 : Subsystem
  gama : Constant  Value=20
  gama_0 : Constant  Value=1.8
  r : Constant  Value=537/18
  segma : Constant  Value=1.65
  Out1 : Outport
  wires:
  Product2/1 -> Product3/1
  K_a/2(Out2) -> Product3/2
  eta_B/1(Out1) -> Add/1
  Product/1 -> Out1/1
  r/1 -> eta_B/2(In2), eta_B0/1(In1)
  gama/1 -> eta_B/1(In1), Beta/1(In1), Product5/2
  Product4/1 -> Product/2
  Constant4/1 -> Product5/1
  Beta/1(Out1) -> Product/1
  Add/1 -> Math Function/1
  Product3/1 -> Math Function1/1
  gama_0/1 -> eta_B0/2(In2)
  Product1/1 -> Product/3
  segma/1 -> Add1/1
  Add1/1 -> Product1/2
  Constant/1 -> Math Function/2
  E_m/1 -> Product2/1
  Math Function/1 -> Product/4
  Constant3/1 -> Product1/1
  K_a/1(Out1) -> Beta/2(In2)
  Product5/1 -> Product4/2
  In2/1 -> K_a/2(In2)
  In1/1 -> K_a/1(In1), Product2/2
  In4/1 -> K_a/3(In3)
  eta_B0/1(Out1) -> Add/2
  Math Function1/1 -> Product/5
  Constant1/1 -> Add1/2, Product4/1

== system Final_System_Model_V10/Full System/Electrolysers/93 KW Electrolyzer Stack_2/electrolyser stack/electrolyser cell/eta_a/m_a ==
  In1 : Inport
  Constant : Constant
  Divide : Product  Inputs=*/
  Subtract : Sum  Inputs=+-
  limiting current : Constant  Value=2
  Out1 : Outport
  wires:
  Divide/1 -> Subtract/2
  Subtract/1 -> Out1/1
  Constant/1 -> Subtract/1
  limiting current/1 -> Divide/2
  In1/1 -> Divide/1

== system Final_System_Model_V10/Full System/Electrolysers/93 KW Electrolyzer Stack_2/electrolyser stack/electrolyser cell/eta_a/n_a ==
  In1 : Inport
  In2 : Inport  Port=2
  In3 : Inport  Port=3
  Divide : Product  Inputs=*/
  i_a0 : Subsystem
  Out1 : Outport
  wires:
  In3/1 -> Divide/1
  In1/1 -> i_a0/2(In2)
  Divide/1 -> Out1/1
  i_a0/1(Out1) -> Divide/2
  In2/1 -> i_a0/1(In1)

== system Final_System_Model_V10/Full System/Electrolysers/93 KW Electrolyzer Stack_2/electrolyser stack/electrolyser cell/eta_c/m_c ==
  In1 : Inport
  Constant : Constant
  Divide : Product  Inputs=*/
  Subtract : Sum  Inputs=+-
  limiting current : Constant  Value=0.00023
  Out1 : Outport
  wires:
  In1/1 -> Divide/1
  Divide/1 -> Subtract/2
  limiting current/1 -> Divide/2
  Subtract/1 -> Out1/1
  Constant/1 -> Subtract/1

== system Final_System_Model_V10/Full System/Electrolysers/93 KW Electrolyzer Stack_2/electrolyser stack/electrolyser cell/eta_c/n_c ==
  In1 : Inport
  In2 : Inport  Port=2
  In3 : Inport  Port=3
  Divide : Product  Inputs=*/
  i_c0 : Subsystem
  Out1 : Outport
  wires:
  In3/1 -> Divide/1
  Divide/1 -> Out1/1
  In1/1 -> i_c0/2(In2)
  i_c0/1(Out1) -> Divide/2
  In2/1 -> i_c0/1(In1)

== system Final_System_Model_V10/Full System/Subsystem1/100KW Fuel Cell Stack_2/Fuel Cell Model/ From Current Density (A//cm^2) To Overvoltages (V)/Concentration Overvoltage/IF Function ==
  In1 : Inport
  Compare To Zero : simulink/Logic and Bit Operations/Compare To Zero  relop=<=  OutDataTypeStr=boolean
  If : If  IfExpression=u1 == 0
  If Action Subsystem : Subsystem  TreatAsAtomicUnit=on
  If Action Subsystem1 : Subsystem  TreatAsAtomicUnit=on
  Merge : Merge  InitialOutput=1
  Out1 : Outport
  wires:
  If Action Subsystem1/1(Out1) -> Merge/2
  Compare To Zero/1 -> If/1
  Merge/1 -> Out1/1
  In1/1 -> If Action Subsystem/1(In1), Compare To Zero/1
  If/2 -> If Action Subsystem1/Action
  If Action Subsystem/1(Out1) -> Merge/1
  If/1 -> If Action Subsystem/Action

== system Final_System_Model_V10/Full System/Subsystem1/100KW Fuel Cell Stack_2/Fuel Cell Model/From Pressures (atm) To Nernest Voltage (V)/From Absolute Pressure (atm) To Partial Pressures (atm)/Hydrogen Partial Pressure Output ==
  note: This block calculates the Hydrogen partial Pressure (pp_H2)(atm)
      | pp_H2 = 0.5 .*((P_H2)./(exp(1.653 .*i./(Tk.^1.334))))-P_H2O
      | where: pp_H2= Hydrogen Partial Pressure (atm)
      | i=Current Density (A/cm^2)
      | Tk= Temperature in Kelvin
      | P_H2O= Water pressure (atm)
  Hydrogen Pressure (P_H2) : Inport
  Temperature/C : Inport  Port=2
  Current Density (i ) : Inport  Port=3
  Water Pressure : Inport  Port=4
  Add : Sum
  Bus Creator : BusCreator  Inputs=6
  Bus Selector : BusSelector  OutputSignals=Stack Temperature (C),273:15,1:653,Current Density (A/cm^2),Hydrogen Pressure (atm),Water Pressure(atm)
  Constant : Constant  Value=273.15
  Constant1 : Constant  Value=1.653
  Constant2 : Constant  Value=1.334
  Divide : Product  Inputs=/*
  Divide1 : Product  Inputs=/*
  Gain : Gain  Gain=0.5
  Math Function : Math  Operator=pow  SaturateOnIntegerOverflow=on
  Math Function1 : Math  SaturateOnIntegerOverflow=on
  Product : Product
  Subtract : Sum  Inputs=+-
  Hydrogen Partial Pressure (pp_H2) : Outport
  wires:
  Water Pressure/1 -> Bus Creator/4
  Temperature/C/1 -> Bus Creator/3
  Current Density (i )/1 -> Bus Creator/2
  Hydrogen Pressure (P_H2)/1 -> Bus Creator/1
  Bus Creator/1 -> Bus Selector/1
  Bus Selector/5 -> Divide1/2  "<Hydrogen Pressure (atm)>"
  Bus Selector/1 -> Add/1  "<Stack Temperature (C)>"
  Constant/1 -> Bus Creator/5  "273:15"
  Add/1 -> Math Function/1  "Temperature/K"
  Constant1/1 -> Bus Creator/6  "1:653"
  Bus Selector/2 -> Add/2  "<273:15>"
  Bus Selector/3 -> Product/1  "<1:653>"
  Bus Selector/4 -> Product/2  "<Current Density (A/cm^2)>"
  Product/1 -> Divide/2
  Divide/1 -> Math Function1/1
  Constant2/1 -> Math Function/2
  Math Function/1 -> Divide/1
  Math Function1/1 -> Divide1/1
  Divide1/1 -> Gain/1
  Bus Selector/6 -> Subtract/2  "<Water Pressure(atm)>"
  Subtract/1 -> Hydrogen Partial Pressure (pp_H2)/1
  Gain/1 -> Subtract/1

== system Final_System_Model_V10/Full System/Subsystem1/100KW Fuel Cell Stack_2/Fuel Cell Model/From Pressures (atm) To Nernest Voltage (V)/From Absolute Pressure (atm) To Partial Pressures (atm)/Oxygen Partial Pressure Output ==
  note: This block calculates the Oxygen Partial Pressure (atm)
      | pp_O2 = (P_air./exp(4.192 .*i/(Tk.^1.334)))-P_H2O
      |
      | where: pp_O2= Oxygen Partial Pressure (atm)
      | P_air= Air Pressure (atm)
      | i= Current Density (A/cm^2)
      | Tk= Temperature (K)
      | P_H2O=Water Pressure (atm)
  Air Pressure (P_air) : Inport
  Temperature/C : Inport  Port=2
  Current Density/i : Inport  Port=3
  Water Pressure : Inport  Port=4
  Add : Sum
  Bus Creator : BusCreator  Inputs=7
  Bus Selector : BusSelector  OutputSignals=Stack Temperature (C),273:15,1:334,Current Density (A/cm^2),4:192,Air Pressure (atm),Water Pressure(atm)
  Constant : Constant  Value=273.15
  Constant1 : Constant  Value=4.192
  Constant2 : Constant  Value=1.334
  Divide : Product  Inputs=/*
  Divide1 : Product  Inputs=/*
  Math Function : Math  Operator=pow  SaturateOnIntegerOverflow=on
  Math Function1 : Math  SaturateOnIntegerOverflow=on
  Product : Product
  Subtract : Sum  Inputs=+-
  Oxygen Partial Pressure pp_O2 : Outport
  wires:
  Current Density/i/1 -> Bus Creator/2
  Water Pressure/1 -> Bus Creator/4
  Temperature/C/1 -> Bus Creator/3
  Air Pressure (P_air)/1 -> Bus Creator/1
  Constant/1 -> Bus Creator/5  "273:15"
  Constant1/1 -> Bus Creator/6  "4:192"
  Constant2/1 -> Bus Creator/7  "1:334"
  Bus Creator/1 -> Bus Selector/1
  Bus Selector/1 -> Add/1  "<Stack Temperature (C)>"
  Bus Selector/2 -> Add/2  "<273:15>"
  Add/1 -> Math Function/1  "Temperature/K"
  Bus Selector/3 -> Math Function/2  "<1:334>"
  Bus Selector/4 -> Product/1  "<Current Density (A/cm^2)>"
  Bus Selector/5 -> Product/2  "<4:192>"
  Product/1 -> Divide/2
  Math Function/1 -> Divide/1
  Divide/1 -> Math Function1/1
  Math Function1/1 -> Divide1/1
  Bus Selector/6 -> Divide1/2  "<Air Pressure (atm)>"
  Divide1/1 -> Subtract/1
  Bus Selector/7 -> Subtract/2  "<Water Pressure(atm)>"
  Subtract/1 -> Oxygen Partial Pressure pp_O2/1  "Oxygen Partial Pressure pp_O2 (atm)"

== system Final_System_Model_V10/Full System/Subsystem1/100KW Fuel Cell Stack_2/Fuel Cell Model/From Pressures (atm) To Nernest Voltage (V)/From Absolute Pressure (atm) To Partial Pressures (atm)/Water Pressure output ==
  note: This block calculates the water saturation Pressure (atm) from the Fuel Cell Temperature (k)
      | x = -2.1794 + 0.02953 .*Tc-9.1837 .*(10.^-5) .*(Tc.^2) + 1.4454 .*(10.^-7) .*(Tc.^3);
      | where: x=Water Saturation Pressure (atm)
      | Tc= Temperature in degree celsius
  Temperature/C : Inport
  -1 : Constant  Value=-7
  -2 : Constant  Value=3
  -5 : Constant  Value=-5
  0.02953 : Constant  Value=0.02953
  0.1 : Constant  Value=9.1837
  0.2 : Constant  Value=1.4454
  Add : Sum  Inputs=+++-
  Constant4 : Constant  Value=-2.1794
  Math Function4 : Math  Operator=10^u  SaturateOnIntegerOverflow=on
  Math Function5 : Math  Operator=square  SaturateOnIntegerOverflow=on
  Math Function6 : Math  Operator=10^u  SaturateOnIntegerOverflow=on
  Math Function7 : Math  Operator=pow  SaturateOnIntegerOverflow=on
  Product1 : Product  Inputs=3
  Product2 : Product
  Product3 : Product  Inputs=3
  "water  pressure " : Math  Operator=10^u  SaturateOnIntegerOverflow=on
  Water Pressure : Outport
  wires:
  Add/1 -> "water  pressure "/1
  0.2/1 -> Product3/1
  Math Function7/1 -> Product3/3
  "water  pressure "/1 -> Water Pressure/1  "Water Pressure(atm)"
  0.02953/1 -> Product2/1
  0.1/1 -> Product1/1
  -5/1 -> Math Function4/1
  Math Function4/1 -> Product1/2
  -1/1 -> Math Function6/1
  Temperature/C/1 -> Product2/2, Math Function5/1, Math Function7/1
  Math Function5/1 -> Product1/3
  -2/1 -> Math Function7/2
  Product2/1 -> Add/2
  Product3/1 -> Add/3
  Math Function6/1 -> Product3/2
  Constant4/1 -> Add/1
  Product1/1 -> Add/4

== system Final_System_Model_V10/Full System/Subsystem1/100KW Fuel Cell Stack_2/Fuel Cell Model/From Pressures (atm) To Nernest Voltage (V)/From Partial Pressures (atm) To Nernest Voltage (V)/IF Function ==
  In1 : Inport
  Constant1 : Constant
  If : If
  If Action Subsystem : Subsystem  TreatAsAtomicUnit=on
  If Action Subsystem1 : Subsystem  TreatAsAtomicUnit=on
  Merge : Merge
  Out1 : Outport
  wires:
  Constant1/1 -> If Action Subsystem1/1(In1)
  If Action Subsystem1/1(Out1) -> Merge/2
  If/1 -> If Action Subsystem/Action
  If/2 -> If Action Subsystem1/Action
  In1/1 -> If Action Subsystem/1(In1), If/1
  Merge/1 -> Out1/1
  If Action Subsystem/1(Out1) -> Merge/1

== system Final_System_Model_V10/Full System/Subsystem1/80KW Fuel Cell Stack_1/Fuel Cell Model/ From Current Density (A//cm^2) To Overvoltages (V)/Concentration Overvoltage/IF Function ==
  In1 : Inport
  Compare To Zero : simulink/Logic and Bit Operations/Compare To Zero  relop=<=  OutDataTypeStr=boolean
  If : If  IfExpression=u1 == 0
  If Action Subsystem : Subsystem  TreatAsAtomicUnit=on
  If Action Subsystem1 : Subsystem  TreatAsAtomicUnit=on
  Merge : Merge  InitialOutput=1
  Out1 : Outport
  wires:
  If/1 -> If Action Subsystem/Action
  If Action Subsystem/1(Out1) -> Merge/1
  If/2 -> If Action Subsystem1/Action
  In1/1 -> Compare To Zero/1, If Action Subsystem/1(In1)
  Merge/1 -> Out1/1
  Compare To Zero/1 -> If/1
  If Action Subsystem1/1(Out1) -> Merge/2

== system Final_System_Model_V10/Full System/Subsystem1/80KW Fuel Cell Stack_1/Fuel Cell Model/From Pressures (atm) To Nernest Voltage (V)/From Absolute Pressure (atm) To Partial Pressures (atm)/Hydrogen Partial Pressure Output ==
  note: This block calculates the Hydrogen partial Pressure (pp_H2)(atm)
      | pp_H2 = 0.5 .*((P_H2)./(exp(1.653 .*i./(Tk.^1.334))))-P_H2O
      | where: pp_H2= Hydrogen Partial Pressure (atm)
      | i=Current Density (A/cm^2)
      | Tk= Temperature in Kelvin
      | P_H2O= Water pressure (atm)
  Hydrogen Pressure (P_H2) : Inport
  Temperature/C : Inport  Port=2
  Current Density (i ) : Inport  Port=3
  Water Pressure : Inport  Port=4
  Add : Sum
  Bus Creator : BusCreator  Inputs=6
  Bus Selector : BusSelector  OutputSignals=Stack Temperature (C),273:15,1:653,Current Density (A/cm^2),Hydrogen Pressure (atm),Water Pressure(atm)
  Constant : Constant  Value=273.15
  Constant1 : Constant  Value=1.653
  Constant2 : Constant  Value=1.334
  Divide : Product  Inputs=/*
  Divide1 : Product  Inputs=/*
  Gain : Gain  Gain=0.5
  Math Function : Math  Operator=pow  SaturateOnIntegerOverflow=on
  Math Function1 : Math  SaturateOnIntegerOverflow=on
  Product : Product
  Subtract : Sum  Inputs=+-
  Hydrogen Partial Pressure (pp_H2) : Outport
  wires:
  Gain/1 -> Subtract/1
  Subtract/1 -> Hydrogen Partial Pressure (pp_H2)/1
  Bus Selector/6 -> Subtract/2  "<Water Pressure(atm)>"
  Divide1/1 -> Gain/1
  Math Function1/1 -> Divide1/1
  Math Function/1 -> Divide/1
  Constant2/1 -> Math Function/2
  Divide/1 -> Math Function1/1
  Product/1 -> Divide/2
  Bus Selector/4 -> Product/2  "<Current Density (A/cm^2)>"
  Bus Selector/3 -> Product/1  "<1:653>"
  Bus Selector/2 -> Add/2  "<273:15>"
  Constant1/1 -> Bus Creator/6  "1:653"
  Add/1 -> Math Function/1  "Temperature/K"
  Constant/1 -> Bus Creator/5  "273:15"
  Bus Selector/1 -> Add/1  "<Stack Temperature (C)>"
  Bus Selector/5 -> Divide1/2  "<Hydrogen Pressure (atm)>"
  Bus Creator/1 -> Bus Selector/1
  Hydrogen Pressure (P_H2)/1 -> Bus Creator/1
  Current Density (i )/1 -> Bus Creator/2
  Temperature/C/1 -> Bus Creator/3
  Water Pressure/1 -> Bus Creator/4

== system Final_System_Model_V10/Full System/Subsystem1/80KW Fuel Cell Stack_1/Fuel Cell Model/From Pressures (atm) To Nernest Voltage (V)/From Absolute Pressure (atm) To Partial Pressures (atm)/Oxygen Partial Pressure Output ==
  note: This block calculates the Oxygen Partial Pressure (atm)
      | pp_O2 = (P_air./exp(4.192 .*i/(Tk.^1.334)))-P_H2O
      |
      | where: pp_O2= Oxygen Partial Pressure (atm)
      | P_air= Air Pressure (atm)
      | i= Current Density (A/cm^2)
      | Tk= Temperature (K)
      | P_H2O=Water Pressure (atm)
  Air Pressure (P_air) : Inport
  Temperature/C : Inport  Port=2
  Current Density/i : Inport  Port=3
  Water Pressure : Inport  Port=4
  Add : Sum
  Bus Creator : BusCreator  Inputs=7
  Bus Selector : BusSelector  OutputSignals=Stack Temperature (C),273:15,1:334,Current Density (A/cm^2),4:192,Air Pressure (atm),Water Pressure(atm)
  Constant : Constant  Value=273.15
  Constant1 : Constant  Value=4.192
  Constant2 : Constant  Value=1.334
  Divide : Product  Inputs=/*
  Divide1 : Product  Inputs=/*
  Math Function : Math  Operator=pow  SaturateOnIntegerOverflow=on
  Math Function1 : Math  SaturateOnIntegerOverflow=on
  Product : Product
  Subtract : Sum  Inputs=+-
  Oxygen Partial Pressure pp_O2 : Outport
  wires:
  Subtract/1 -> Oxygen Partial Pressure pp_O2/1  "Oxygen Partial Pressure pp_O2 (atm)"
  Bus Selector/7 -> Subtract/2  "<Water Pressure(atm)>"
  Divide1/1 -> Subtract/1
  Bus Selector/6 -> Divide1/2  "<Air Pressure (atm)>"
  Math Function1/1 -> Divide1/1
  Divide/1 -> Math Function1/1
  Math Function/1 -> Divide/1
  Product/1 -> Divide/2
  Bus Selector/5 -> Product/2  "<4:192>"
  Bus Selector/4 -> Product/1  "<Current Density (A/cm^2)>"
  Bus Selector/3 -> Math Function/2  "<1:334>"
  Add/1 -> Math Function/1  "Temperature/K"
  Bus Selector/2 -> Add/2  "<273:15>"
  Bus Selector/1 -> Add/1  "<Stack Temperature (C)>"
  Bus Creator/1 -> Bus Selector/1
  Constant2/1 -> Bus Creator/7  "1:334"
  Constant1/1 -> Bus Creator/6  "4:192"
  Constant/1 -> Bus Creator/5  "273:15"
  Air Pressure (P_air)/1 -> Bus Creator/1
  Temperature/C/1 -> Bus Creator/3
  Water Pressure/1 -> Bus Creator/4
  Current Density/i/1 -> Bus Creator/2

== system Final_System_Model_V10/Full System/Subsystem1/80KW Fuel Cell Stack_1/Fuel Cell Model/From Pressures (atm) To Nernest Voltage (V)/From Absolute Pressure (atm) To Partial Pressures (atm)/Water Pressure output ==
  note: This block calculates the water saturation Pressure (atm) from the Fuel Cell Temperature (k)
      | x = -2.1794 + 0.02953 .*Tc-9.1837 .*(10.^-5) .*(Tc.^2) + 1.4454 .*(10.^-7) .*(Tc.^3);
      | where: x=Water Saturation Pressure (atm)
      | Tc= Temperature in degree celsius
  Temperature/C : Inport
  -1 : Constant  Value=-7
  -2 : Constant  Value=3
  -5 : Constant  Value=-5
  0.02953 : Constant  Value=0.02953
  0.1 : Constant  Value=9.1837
  0.2 : Constant  Value=1.4454
  Add : Sum  Inputs=+++-
  Constant4 : Constant  Value=-2.1794
  Math Function4 : Math  Operator=10^u  SaturateOnIntegerOverflow=on
  Math Function5 : Math  Operator=square  SaturateOnIntegerOverflow=on
  Math Function6 : Math  Operator=10^u  SaturateOnIntegerOverflow=on
  Math Function7 : Math  Operator=pow  SaturateOnIntegerOverflow=on
  Product1 : Product  Inputs=3
  Product2 : Product
  Product3 : Product  Inputs=3
  "water  pressure " : Math  Operator=10^u  SaturateOnIntegerOverflow=on
  Water Pressure : Outport
  wires:
  Product1/1 -> Add/4
  Constant4/1 -> Add/1
  Math Function6/1 -> Product3/2
  Product3/1 -> Add/3
  Product2/1 -> Add/2
  -2/1 -> Math Function7/2
  Math Function5/1 -> Product1/3
  Temperature/C/1 -> Math Function7/1, Math Function5/1, Product2/2
  -1/1 -> Math Function6/1
  Math Function4/1 -> Product1/2
  -5/1 -> Math Function4/1
  0.1/1 -> Product1/1
  0.02953/1 -> Product2/1
  "water  pressure "/1 -> Water Pressure/1  "Water Pressure(atm)"
  Math Function7/1 -> Product3/3
  0.2/1 -> Product3/1
  Add/1 -> "water  pressure "/1

== system Final_System_Model_V10/Full System/Subsystem1/80KW Fuel Cell Stack_1/Fuel Cell Model/From Pressures (atm) To Nernest Voltage (V)/From Partial Pressures (atm) To Nernest Voltage (V)/IF Function ==
  In1 : Inport
  Constant1 : Constant
  If : If
  If Action Subsystem : Subsystem  TreatAsAtomicUnit=on
  If Action Subsystem1 : Subsystem  TreatAsAtomicUnit=on
  Merge : Merge
  Out1 : Outport
  wires:
  If Action Subsystem/1(Out1) -> Merge/1
  Merge/1 -> Out1/1
  In1/1 -> If/1, If Action Subsystem/1(In1)
  If/2 -> If Action Subsystem1/Action
  If/1 -> If Action Subsystem/Action
  If Action Subsystem1/1(Out1) -> Merge/2
  Constant1/1 -> If Action Subsystem1/1(In1)
